simulink model "AcO_Ctrl_Geometric_headless_R2016a"  (R2016a)
settings: Solver=FixedStepDiscrete  StartTime=0.0  StopTime=simulation_duration  FixedStep=Ts  RelTol=1e-3
values from neighbouring files (symbols this model uses):
  M1_BeMo_d = zeros(7,M1_n_mode)    [AcO_Ctrl_headless_cfg.m]    (also in agws_cfg.m = 1e-6*bsxfun(@times,randn(7,M1_n_mode),scale); agws_fastTT_cfg.m = 1e-6*bsxfun(@times,randn(7,M1_n_mode),scale))
  M1_RiBo_d = zeros(7,6)    [AcO_Ctrl_headless_cfg.m]    (also in agws_cfg.m = [M1_Txyz0 M1_Rxyz0]; agws_fastTT_cfg.m = [M1_Txyz0 M1_Rxyz0])
  M2_RiBo_d = zeros(7,6)    [AcO_Ctrl_headless_cfg.m]    (also in agws_cfg.m = [M2_Txyz0 M2_Rxyz0]; agws_fastTT_cfg.m = [M2_Txyz0 M2_Rxyz0])
  Ts = 1/fs    (= 0.002)    [AcO_Ctrl_headless_cfg.m]    (also in agws_fastTT_cfg.m = 0.005)
undefined symbols (not defined in the file or in its folder): Az_C, CG2Hp, CG2Hp_S7, El_C, Fsmm, GIR_C, Hp2CG_f, Hp2CG_f_S7, HPdtf, HpK, KM2, M2_actdyn, M2_CG2Hp, M_LOS, MIMO_C, PTT2act, PTT2act_even, Q, sysd, TT2act, TT2act_even
undefined symbols (not defined in the file): on_axis_src_outputs
libraries: CEO x2
(part 3 of 6)

== system AcO_Ctrl_Geometric_headless_R2016a/Structural Dynamics V3.3/Structural Dynamics V3.3/Structural Dynamics Plus CL Az El M1 force/Az Control ==
  In1 : Inport
  -1(2) : Gain  Gain=-ones(4,1)  Multiplication=Matrix(K*u)
  Azimuth Controller : DiscreteFilter  Numerator=Az_C.num{1}  Denominator=Az_C.den{1}  SampleTime=1/500
  DEMUX1 : Gain  Gain=ones(4,1)  Multiplication=Matrix(K*u)
  Out1 : Outport
  Out2 : Outport  Port=2
  wires:
  -1(2)/1 -> Out2/1
  Azimuth Controller/1 -> DEMUX1/1, -1(2)/1
  DEMUX1/1 -> Out1/1
  In1/1 -> Azimuth Controller/1

== system AcO_Ctrl_Geometric_headless_R2016a/Structural Dynamics V3.3/Structural Dynamics V3.3/Structural Dynamics Plus CL Az El M1 force/Az El Sensing ==
  note: Note: units are m, not radians for these loops!
      | These loops delta the top and bottom displacements in tangential direction, and average the results.
  Az_top_disp(4) : Inport
  El_bottom_disp(4) : Inport  Port=2
  El_top_disp(4) : Inport  Port=3
  Az_bot_disp(4) : Inport  Port=4
  Az : Scope
  El : Scope
  Sum2 : Sum  Inputs=-+|
  Sum3 : Sum  Inputs=-+|
  average : Gain  Gain=ones(1,4)/4  Multiplication=Matrix(K*u)
  average1 : Gain  Gain=ones(1,4)/4  Multiplication=Matrix(K*u)
  El_average(1) : Outport
  Az_average(1) : Outport  Port=2
  wires:
  El_top_disp(4)/1 -> Sum2/2
  El_bottom_disp(4)/1 -> Sum2/1
  Sum2/1 -> average/1
  Sum3/1 -> average1/1
  average1/1 -> Az/1, Az_average(1)/1
  Az_bot_disp(4)/1 -> Sum3/1
  Az_top_disp(4)/1 -> Sum3/2
  average/1 -> El_average(1)/1, El/1

== system AcO_Ctrl_Geometric_headless_R2016a/Structural Dynamics V3.3/Structural Dynamics V3.3/Structural Dynamics Plus CL Az El M1 force/El Control ==
  In1 : Inport
  -1 : Gain  Gain=-ones(4,1)  Multiplication=Matrix(K*u)
  DEMUX : Gain  Gain=ones(4,1)  Multiplication=Matrix(K*u)
  Elevation Controller : DiscreteFilter  Numerator=El_C.num{1}  Denominator=El_C.den{1}  SampleTime=1/500
  Out1 : Outport
  Out2 : Outport  Port=2
  wires:
  In1/1 -> Elevation Controller/1
  DEMUX/1 -> Out2/1
  -1/1 -> Out1/1
  Elevation Controller/1 -> DEMUX/1, -1/1

== system AcO_Ctrl_Geometric_headless_R2016a/Structural Dynamics V3.3/Structural Dynamics V3.3/Structural Dynamics Plus CL Az El M1 force/M1 Displacement Local Control ==
  note: Offset displacement, used
      | in calcuation of hard point
      | forces.
  note: Hexapod Offset Forces
  note: Hexapod Desired Lengths
  note: This block converts from CG displacements and rotations,
      | and converts to Hard Point lengths.  Hard point lengths are
      | changed by applying an equal and opposite force to the hard
      | point, and then offseting output by the commanded change
      | in position.
  note: CG desired displacement/rotation
  M1_cmd(42) : Inport
  CG2Hp{1..6} (6 alike) : Gain  Gain=CG2Hp  Multiplication=Matrix(K*u)
  CG2Hp7 : Gain  Gain=CG2Hp_S7  Multiplication=Matrix(K*u)
  Demux1 : Demux  Outputs=6*ones(7,1)
  HpK{1,3..8} (7 alike) : Gain  Gain=HpK  Multiplication=Matrix(K*u)
  Mux1 : Mux  Inputs=6*ones(7,1)
  Mux3 : Mux  Inputs=6*ones(7,1)
  M1_HP_D_cmd(42) : Outport
  M1_HP_F_cmd (42) : Outport  Port=2
  wires:
  HpK8/1 -> Mux3/1
  CG2Hp7/1 -> Mux1/1, HpK8/1
  Demux1/1 -> CG2Hp7/1
  Demux1/7 -> CG2Hp6/1
  Demux1/6 -> CG2Hp5/1
  Demux1/5 -> CG2Hp4/1
  Demux1/4 -> CG2Hp3/1
  Demux1/3 -> CG2Hp2/1
  HpK7/1 -> Mux3/7
  HpK6/1 -> Mux3/6
  HpK5/1 -> Mux3/5
  HpK4/1 -> Mux3/4
  HpK1/1 -> Mux3/3
  CG2Hp6/1 -> HpK7/1, Mux1/7
  CG2Hp5/1 -> HpK6/1, Mux1/6
  CG2Hp4/1 -> HpK5/1, Mux1/5
  CG2Hp3/1 -> HpK4/1, Mux1/4
  CG2Hp2/1 -> Mux1/3, HpK1/1
  CG2Hp1/1 -> HpK3/1, Mux1/2
  Demux1/2 -> CG2Hp1/1
  M1_cmd(42)/1 -> Demux1/1
  Mux1/1 -> M1_HP_D_cmd(42)/1
  Mux3/1 -> M1_HP_F_cmd (42)/1
  HpK3/1 -> Mux3/2

== system AcO_Ctrl_Geometric_headless_R2016a/Structural Dynamics V3.3/Structural Dynamics V3.3/Structural Dynamics Plus CL Az El M1 force/M1 Force Control ==
  note: Face Forces (N)
  note: Cell Forces (N)
  note: in Newtons
  M1_measured_Force(42) : Inport
  ControlM1S1 : Subsystem
  ControlM1S2 : Subsystem
  ControlM1S3 : Subsystem
  ControlM1S4 : Subsystem
  ControlM1S5 : Subsystem
  ControlM1S6 : Subsystem
  ControlM1S7 : Subsystem
  Demux3 : Demux  Outputs=6*ones(7,1)
  M1S7 FaceForce : Outport
  M1S1 FaceForce : Outport  Port=2
  M1S2 FaceForce : Outport  Port=3
  M1S3 FaceForce : Outport  Port=4
  M1S4 FaceForce : Outport  Port=5
  M1S5 FaceForce : Outport  Port=6
  M1S6 FaceForce : Outport  Port=7
  M1S7 CellForce : Outport  Port=8
  M1S1 CellForce : Outport  Port=9
  M1S2 CellForce : Outport  Port=10
  M1S3 CellForce : Outport  Port=11
  M1S4 CellForce : Outport  Port=12
  M1S5 CellForce : Outport  Port=13
  M1S6 CellForce : Outport  Port=14
  wires:
  ControlM1S7/2(Out2) -> M1S7 CellForce/1
  ControlM1S7/1(Out1) -> M1S7 FaceForce/1
  Demux3/1 -> ControlM1S7/1(In1)
  ControlM1S6/2(Out2) -> M1S6 CellForce/1
  ControlM1S5/2(Out2) -> M1S5 CellForce/1
  ControlM1S4/2(Out2) -> M1S4 CellForce/1
  ControlM1S3/2(Out2) -> M1S3 CellForce/1
  ControlM1S2/2(Out2) -> M1S2 CellForce/1
  ControlM1S6/1(Out1) -> M1S6 FaceForce/1
  ControlM1S5/1(Out1) -> M1S5 FaceForce/1
  ControlM1S4/1(Out1) -> M1S4 FaceForce/1
  ControlM1S3/1(Out1) -> M1S3 FaceForce/1
  ControlM1S2/1(Out1) -> M1S2 FaceForce/1
  Demux3/7 -> ControlM1S6/1(In1)
  Demux3/6 -> ControlM1S5/1(In1)
  Demux3/5 -> ControlM1S4/1(In1)
  Demux3/4 -> ControlM1S3/1(In1)
  Demux3/3 -> ControlM1S2/1(In1)
  Demux3/2 -> ControlM1S1/1(In1)
  ControlM1S1/1(Out1) -> M1S1 FaceForce/1
  ControlM1S1/2(Out2) -> M1S1 CellForce/1
  M1_measured_Force(42)/1 -> Demux3/1

== system AcO_Ctrl_Geometric_headless_R2016a/Structural Dynamics V3.3/Structural Dynamics V3.3/Structural Dynamics Plus CL Az El M1 force/M1 Sensing ==
  M1_cmd (42) : Inport
  M1_HP_cell(42) : Inport  Port=2
  M1_HPface(42) : Inport  Port=3
  Demux1 : Demux  Outputs=6*ones(7,1)
  Demux2 : Demux  Outputs=6*ones(7,1)
  Demux9 : Demux  Outputs=6*ones(7,1)
  Mux3 : Mux  Inputs=6*ones(7,1)
  Scope : Scope
  Scope1 : Scope
  senseM1S1 : Subsystem
  senseM1S2 : Subsystem
  senseM1S3 : Subsystem
  senseM1S4 : Subsystem
  senseM1S5 : Subsystem
  senseM1S6 : Subsystem
  senseM1S7 : Subsystem
  M1 Hard Point Force(42) : Outport
  wires:
  M1_HPface(42)/1 -> Demux1/1
  Demux9/7 -> senseM1S6/1(HP_D_cmd)
  Demux9/5 -> senseM1S4/1(HP_D_cmd)
  Demux9/1 -> senseM1S7/1(HP_D_cmd)
  Demux9/6 -> senseM1S5/1(HP_D_cmd)
  Demux9/4 -> senseM1S3/1(HP_D_cmd)
  M1_cmd (42)/1 -> Demux9/1
  Demux9/3 -> senseM1S2/1(HP_D_cmd)
  Demux1/3 -> senseM1S2/2(HP_D_face)
  Demux1/2 -> senseM1S1/2(HP_D_face), Scope1/1
  Demux9/2 -> senseM1S1/1(HP_D_cmd)
  Mux3/1 -> M1 Hard Point Force(42)/1
  senseM1S6/1(HardPoint_6DOF_Force) -> Mux3/7
  Demux1/6 -> senseM1S5/2(HP_D_face)
  Demux1/7 -> senseM1S6/2(HP_D_face)
  Demux2/1 -> senseM1S7/3(HP_D_cell)
  M1_HP_cell(42)/1 -> Demux2/1
  senseM1S2/1(HardPoint_6DOF_Force) -> Mux3/3
  senseM1S3/1(HardPoint_6DOF_Force) -> Mux3/4
  senseM1S4/1(HardPoint_6DOF_Force) -> Mux3/5
  Demux1/1 -> senseM1S7/2(HP_D_face)
  Demux2/6 -> senseM1S5/3(HP_D_cell)
  Demux2/7 -> senseM1S6/3(HP_D_cell)
  senseM1S7/1(HardPoint_6DOF_Force) -> Mux3/1
  senseM1S5/1(HardPoint_6DOF_Force) -> Mux3/6
  Demux1/5 -> senseM1S4/2(HP_D_face)
  Demux2/4 -> senseM1S3/3(HP_D_cell)
  Demux2/3 -> senseM1S2/3(HP_D_cell)
  Demux2/2 -> senseM1S1/3(HP_D_cell)
  senseM1S1/1(HardPoint_6DOF_Force) -> Mux3/2, Scope/1
  Demux1/4 -> senseM1S3/2(HP_D_face)
  Demux2/5 -> senseM1S4/3(HP_D_cell)

== system AcO_Ctrl_Geometric_headless_R2016a/Structural Dynamics V3.3/Structural Dynamics V3.3/Structural Dynamics Plus CL Az El M1 force/M2 control ==
  note: fancy way of outputting equal and opposite forces
  note: TT command (radians)
  note: This one is grouped differently so that it is clear that odds and evens are slightly different.
      | Each subsystem controller includes both the TT controller from TT command, to PZT position command, to PZT force (using an open loop approximation).
  note: in radians
  note: in Newtons
  note: Convert from PTT to actuator
      | DOF
  note: M2 actuator Dynamics
  PTT ref (21) : Inport
  Demux1 : Demux  Outputs=3*ones(7,1)
  M2actuatorDyanmics{1..7} (7 alike) : DiscreteStateSpace  A=M2_actdyn.A  B=M2_actdyn.B  C=M2_actdyn.C  D=M2_actdyn.D  SampleTime=1/Fsmm
  TT_to_act{,1..3} (4 alike) : Gain  Gain=PTT2act  Multiplication=Matrix(K*u)
  TT_to_act4 : Gain  Gain=PTT2act_even  Multiplication=Matrix(K*u)
  TT_to_act5 : Gain  Gain=PTT2act_even  Multiplication=Matrix(K*u)
  TT_to_act6 : Gain  Gain=PTT2act_even  Multiplication=Matrix(K*u)
  delta{2..8} (7 alike) : Gain  Gain=[eye(3);-eye(3)]  Multiplication=Matrix(K*u)
  M2S7PZT_F : Outport
  M2S1PZT_F : Outport  Port=2
  M2S2PZT_F : Outport  Port=3
  M2S3PZT_F : Outport  Port=4
  M2S4PZT_F : Outport  Port=5
  M2S5PZT_F : Outport  Port=6
  M2S6PZT_F : Outport  Port=7
  wires:
  PTT ref (21)/1 -> Demux1/1
  delta5/1 -> M2S3PZT_F/1
  delta3/1 -> M2S1PZT_F/1
  TT_to_act6/1 -> M2actuatorDyanmics7/1
  M2actuatorDyanmics7/1 -> delta8/1
  TT_to_act3/1 -> M2actuatorDyanmics6/1
  M2actuatorDyanmics6/1 -> delta7/1
  TT_to_act5/1 -> M2actuatorDyanmics5/1
  M2actuatorDyanmics5/1 -> delta6/1
  TT_to_act2/1 -> M2actuatorDyanmics4/1
  M2actuatorDyanmics4/1 -> delta5/1
  TT_to_act4/1 -> M2actuatorDyanmics3/1
  M2actuatorDyanmics3/1 -> delta4/1
  TT_to_act1/1 -> M2actuatorDyanmics2/1
  M2actuatorDyanmics2/1 -> delta3/1
  TT_to_act/1 -> M2actuatorDyanmics1/1
  M2actuatorDyanmics1/1 -> delta2/1
  delta8/1 -> M2S6PZT_F/1
  delta7/1 -> M2S5PZT_F/1
  delta6/1 -> M2S4PZT_F/1
  delta4/1 -> M2S2PZT_F/1
  delta2/1 -> M2S7PZT_F/1
  Demux1/1 -> TT_to_act/1
  Demux1/7 -> TT_to_act6/1
  Demux1/6 -> TT_to_act3/1
  Demux1/5 -> TT_to_act5/1
  Demux1/4 -> TT_to_act2/1
  Demux1/3 -> TT_to_act4/1
  Demux1/2 -> TT_to_act1/1

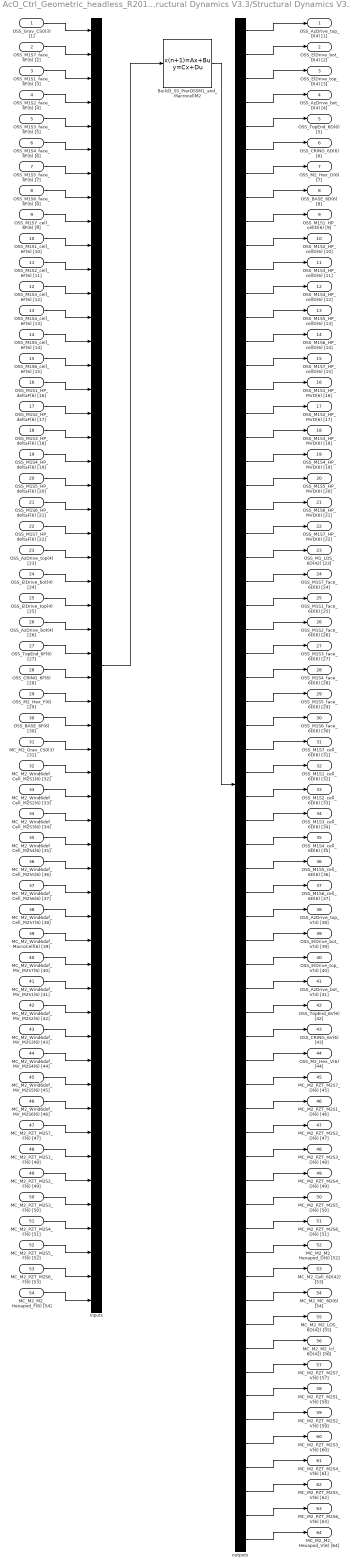
== system AcO_Ctrl_Geometric_headless_R2016a/Structural Dynamics V3.3/Structural Dynamics V3.3/Structural Dynamics Plus CL Az El M1 force/PlantDynamics Build3_SS_PierOSSM1_and_MacrocellM2 ==
  OSS_Grav_CS0(3) [1] : Inport  PortDimensions=3
  OSS_M1S7_face_6F(6) [2] : Inport  Port=2  PortDimensions=6
  OSS_M1S1_face_6F(6) [3] : Inport  Port=3  PortDimensions=6
  OSS_M1S2_face_6F(6) [4] : Inport  Port=4  PortDimensions=6
  OSS_M1S3_face_6F(6) [5] : Inport  Port=5  PortDimensions=6
  OSS_M1S4_face_6F(6) [6] : Inport  Port=6  PortDimensions=6
  OSS_M1S5_face_6F(6) [7] : Inport  Port=7  PortDimensions=6
  OSS_M1S6_face_6F(6) [8] : Inport  Port=8  PortDimensions=6
  OSS_M1S7_cell_6F(6) [9] : Inport  Port=9  PortDimensions=6
  OSS_M1S1_cell_6F(6) [10] : Inport  Port=10  PortDimensions=6
  OSS_M1S2_cell_6F(6) [11] : Inport  Port=11  PortDimensions=6
  OSS_M1S3_cell_6F(6) [12] : Inport  Port=12  PortDimensions=6
  OSS_M1S4_cell_6F(6) [13] : Inport  Port=13  PortDimensions=6
  OSS_M1S5_cell_6F(6) [14] : Inport  Port=14  PortDimensions=6
  OSS_M1S6_cell_6F(6) [15] : Inport  Port=15  PortDimensions=6
  OSS_M1S1_HP_deltaF(6) [16] : Inport  Port=16  PortDimensions=6
  OSS_M1S2_HP_deltaF(6) [17] : Inport  Port=17  PortDimensions=6
  OSS_M1S3_HP_deltaF(6) [18] : Inport  Port=18  PortDimensions=6
  OSS_M1S4_HP_deltaF(6) [19] : Inport  Port=19  PortDimensions=6
  OSS_M1S5_HP_deltaF(6) [20] : Inport  Port=20  PortDimensions=6
  OSS_M1S6_HP_deltaF(6) [21] : Inport  Port=21  PortDimensions=6
  OSS_M1S7_HP_deltaF(6) [22] : Inport  Port=22  PortDimensions=6
  OSS_AzDrive_top(4) [23] : Inport  Port=23  PortDimensions=4
  OSS_ElDrive_bot(4) [24] : Inport  Port=24  PortDimensions=4
  OSS_ElDrive_top(4) [25] : Inport  Port=25  PortDimensions=4
  OSS_AzDrive_bot(4) [26] : Inport  Port=26  PortDimensions=4
  OSS_TopEnd_6F(6) [27] : Inport  Port=27  PortDimensions=6
  OSS_CRING_6F(6) [28] : Inport  Port=28  PortDimensions=6
  OSS_M2_Hex_F(6) [29] : Inport  Port=29  PortDimensions=6
  OSS_BASE_6F(6) [30] : Inport  Port=30  PortDimensions=6
  MC_M2_Grav_CS0(3) [31] : Inport  Port=31  PortDimensions=3
  MC_M2_Wind6dof_Cell_M2S1(6) [32] : Inport  Port=32  PortDimensions=6
  MC_M2_Wind6dof_Cell_M2S2(6) [33] : Inport  Port=33  PortDimensions=6
  MC_M2_Wind6dof_Cell_M2S3(6) [34] : Inport  Port=34  PortDimensions=6
  MC_M2_Wind6dof_Cell_M2S4(6) [35] : Inport  Port=35  PortDimensions=6
  MC_M2_Wind6dof_Cell_M2S5(6) [36] : Inport  Port=36  PortDimensions=6
  MC_M2_Wind6dof_Cell_M2S6(6) [37] : Inport  Port=37  PortDimensions=6
  MC_M2_Wind6dof_Cell_M2S7(6) [38] : Inport  Port=38  PortDimensions=6
  MC_M2_Wind6dof_MacroCell(6) [39] : Inport  Port=39  PortDimensions=6
  MC_M2_Wind6dof_Mir_M2S7(6) [40] : Inport  Port=40  PortDimensions=6
  MC_M2_Wind6dof_Mir_M2S1(6) [41] : Inport  Port=41  PortDimensions=6
  MC_M2_Wind6dof_Mir_M2S2(6) [42] : Inport  Port=42  PortDimensions=6
  MC_M2_Wind6dof_Mir_M2S3(6) [43] : Inport  Port=43  PortDimensions=6
  MC_M2_Wind6dof_Mir_M2S4(6) [44] : Inport  Port=44  PortDimensions=6
  MC_M2_Wind6dof_Mir_M2S5(6) [45] : Inport  Port=45  PortDimensions=6
  MC_M2_Wind6dof_Mir_M2S6(6) [46] : Inport  Port=46  PortDimensions=6
  MC_M2_PZT_M2S7_F(6) [47] : Inport  Port=47  PortDimensions=6
  MC_M2_PZT_M2S1_F(6) [48] : Inport  Port=48  PortDimensions=6
  MC_M2_PZT_M2S2_F(6) [49] : Inport  Port=49  PortDimensions=6
  MC_M2_PZT_M2S3_F(6) [50] : Inport  Port=50  PortDimensions=6
  MC_M2_PZT_M2S4_F(6) [51] : Inport  Port=51  PortDimensions=6
  MC_M2_PZT_M2S5_F(6) [52] : Inport  Port=52  PortDimensions=6
  MC_M2_PZT_M2S6_F(6) [53] : Inport  Port=53  PortDimensions=6
  MC_M2_M2_Hexapod_F(6) [54] : Inport  Port=54  PortDimensions=6
  Build3_SS_PierOSSM1_and_MacrocellM2 : DiscreteStateSpace  A=sysd.sys.A  B=sysd.sys.B  C=sysd.sys.C  D=sysd.sys.D  SampleTime=0.002
  inputs : Mux  Inputs=[3,6,6,6,6,6,6,6,6,6,6,6,6,6,6,6,6,6,6,6,6,6,4,4,4,4,6,6,6,6,3,6,6,6,6,6,6,6,6,6,6,6,6,6,6,6,6,6,6,6,6,6,6,6]
  outputs : Demux  Outputs=[4,4,4,4,6,6,6,6,6,6,6,6,6,6,6,6,6,6,6,6,6,6,42,6,6,6,6,6,6,6,6,6,6,6,6,6,6,4,4,4,4,6,6,6,6,6,6,6,6,6,6,6,42,6,42,42,6,6,6,6,6,6,6,6]
  OSS_AzDrive_top_D(4) [1] : Outport  PortDimensions=4
  OSS_ElDrive_bot_D(4) [2] : Outport  Port=2  PortDimensions=4
  OSS_ElDrive_top_D(4) [3] : Outport  Port=3  PortDimensions=4
  OSS_AzDrive_bot_D(4) [4] : Outport  Port=4  PortDimensions=4
  OSS_TopEnd_6D(6) [5] : Outport  Port=5  PortDimensions=6
  OSS_CRING_6D(6) [6] : Outport  Port=6  PortDimensions=6
  OSS_M2_Hex_D(6) [7] : Outport  Port=7  PortDimensions=6
  OSS_BASE_6D(6) [8] : Outport  Port=8  PortDimensions=6
  OSS_M1S1_HP_cellD(6) [9] : Outport  Port=9  PortDimensions=6
  OSS_M1S2_HP_cellD(6) [10] : Outport  Port=10  PortDimensions=6
  OSS_M1S3_HP_cellD(6) [11] : Outport  Port=11  PortDimensions=6
  OSS_M1S4_HP_cellD(6) [12] : Outport  Port=12  PortDimensions=6
  OSS_M1S5_HP_cellD(6) [13] : Outport  Port=13  PortDimensions=6
  OSS_M1S6_HP_cellD(6) [14] : Outport  Port=14  PortDimensions=6
  OSS_M1S7_HP_cellD(6) [15] : Outport  Port=15  PortDimensions=6
  OSS_M1S1_HP_MirD(6) [16] : Outport  Port=16  PortDimensions=6
  OSS_M1S2_HP_MirD(6) [17] : Outport  Port=17  PortDimensions=6
  OSS_M1S3_HP_MirD(6) [18] : Outport  Port=18  PortDimensions=6
  OSS_M1S4_HP_MirD(6) [19] : Outport  Port=19  PortDimensions=6
  OSS_M1S5_HP_MirD(6) [20] : Outport  Port=20  PortDimensions=6
  OSS_M1S6_HP_MirD(6) [21] : Outport  Port=21  PortDimensions=6
  OSS_M1S7_HP_MirD(6) [22] : Outport  Port=22  PortDimensions=6
  OSS_M1_LOS_6D(42) [23] : Outport  Port=23  PortDimensions=42
  OSS_M1S7_face_6D(6) [24] : Outport  Port=24  PortDimensions=6
  OSS_M1S1_face_6D(6) [25] : Outport  Port=25  PortDimensions=6
  OSS_M1S2_face_6D(6) [26] : Outport  Port=26  PortDimensions=6
  OSS_M1S3_face_6D(6) [27] : Outport  Port=27  PortDimensions=6
  OSS_M1S4_face_6D(6) [28] : Outport  Port=28  PortDimensions=6
  OSS_M1S5_face_6D(6) [29] : Outport  Port=29  PortDimensions=6
  OSS_M1S6_face_6D(6) [30] : Outport  Port=30  PortDimensions=6
  OSS_M1S7_cell_6D(6) [31] : Outport  Port=31  PortDimensions=6
  OSS_M1S1_cell_6D(6) [32] : Outport  Port=32  PortDimensions=6
  OSS_M1S2_cell_6D(6) [33] : Outport  Port=33  PortDimensions=6
  OSS_M1S3_cell_6D(6) [34] : Outport  Port=34  PortDimensions=6
  OSS_M1S4_cell_6D(6) [35] : Outport  Port=35  PortDimensions=6
  OSS_M1S5_cell_6D(6) [36] : Outport  Port=36  PortDimensions=6
  OSS_M1S6_cell_6D(6) [37] : Outport  Port=37  PortDimensions=6
  OSS_AzDrive_top_V(4) [38] : Outport  Port=38  PortDimensions=4
  OSS_ElDrive_bot_V(4) [39] : Outport  Port=39  PortDimensions=4
  OSS_ElDrive_top_V(4) [40] : Outport  Port=40  PortDimensions=4
  OSS_AzDrive_bot_V(4) [41] : Outport  Port=41  PortDimensions=4
  OSS_TopEnd_6V(6) [42] : Outport  Port=42  PortDimensions=6
  OSS_CRING_6V(6) [43] : Outport  Port=43  PortDimensions=6
  OSS_M2_Hex_V(6) [44] : Outport  Port=44  PortDimensions=6
  MC_M2_PZT_M2S7_D(6) [45] : Outport  Port=45  PortDimensions=6
  MC_M2_PZT_M2S1_D(6) [46] : Outport  Port=46  PortDimensions=6
  MC_M2_PZT_M2S2_D(6) [47] : Outport  Port=47  PortDimensions=6
  MC_M2_PZT_M2S3_D(6) [48] : Outport  Port=48  PortDimensions=6
  MC_M2_PZT_M2S4_D(6) [49] : Outport  Port=49  PortDimensions=6
  MC_M2_PZT_M2S5_D(6) [50] : Outport  Port=50  PortDimensions=6
  MC_M2_PZT_M2S6_D(6) [51] : Outport  Port=51  PortDimensions=6
  MC_M2_M2_Hexapod_D(6) [52] : Outport  Port=52  PortDimensions=6
  MC_M2_Cell_6D(42) [53] : Outport  Port=53  PortDimensions=42
  MC_M2_MC_6D(6) [54] : Outport  Port=54  PortDimensions=6
  MC_M2_M2_LOS_6D(42) [55] : Outport  Port=55  PortDimensions=42
  MC_M2_M2_lcl_6D(42) [56] : Outport  Port=56  PortDimensions=42
  MC_M2_PZT_M2S7_V(6) [57] : Outport  Port=57  PortDimensions=6
  MC_M2_PZT_M2S1_V(6) [58] : Outport  Port=58  PortDimensions=6
  MC_M2_PZT_M2S2_V(6) [59] : Outport  Port=59  PortDimensions=6
  MC_M2_PZT_M2S3_V(6) [60] : Outport  Port=60  PortDimensions=6
  MC_M2_PZT_M2S4_V(6) [61] : Outport  Port=61  PortDimensions=6
  MC_M2_PZT_M2S5_V(6) [62] : Outport  Port=62  PortDimensions=6
  MC_M2_PZT_M2S6_V(6) [63] : Outport  Port=63  PortDimensions=6
  MC_M2_M2_Hexapod_V(6) [64] : Outport  Port=64  PortDimensions=6
  wires:
  outputs/64 -> MC_M2_M2_Hexapod_V(6) [64]/1
  outputs/63 -> MC_M2_PZT_M2S6_V(6) [63]/1
  outputs/62 -> MC_M2_PZT_M2S5_V(6) [62]/1
  outputs/61 -> MC_M2_PZT_M2S4_V(6) [61]/1
  outputs/60 -> MC_M2_PZT_M2S3_V(6) [60]/1
  outputs/59 -> MC_M2_PZT_M2S2_V(6) [59]/1
  outputs/58 -> MC_M2_PZT_M2S1_V(6) [58]/1
  outputs/57 -> MC_M2_PZT_M2S7_V(6) [57]/1
  outputs/56 -> MC_M2_M2_lcl_6D(42) [56]/1
  outputs/55 -> MC_M2_M2_LOS_6D(42) [55]/1
  outputs/54 -> MC_M2_MC_6D(6) [54]/1
  outputs/53 -> MC_M2_Cell_6D(42) [53]/1
  outputs/52 -> MC_M2_M2_Hexapod_D(6) [52]/1
  outputs/51 -> MC_M2_PZT_M2S6_D(6) [51]/1
  outputs/50 -> MC_M2_PZT_M2S5_D(6) [50]/1
  outputs/49 -> MC_M2_PZT_M2S4_D(6) [49]/1
  outputs/48 -> MC_M2_PZT_M2S3_D(6) [48]/1
  outputs/47 -> MC_M2_PZT_M2S2_D(6) [47]/1
  outputs/46 -> MC_M2_PZT_M2S1_D(6) [46]/1
  outputs/45 -> MC_M2_PZT_M2S7_D(6) [45]/1
  outputs/44 -> OSS_M2_Hex_V(6) [44]/1
  outputs/43 -> OSS_CRING_6V(6) [43]/1
  outputs/42 -> OSS_TopEnd_6V(6) [42]/1
  outputs/41 -> OSS_AzDrive_bot_V(4) [41]/1
  outputs/40 -> OSS_ElDrive_top_V(4) [40]/1
  outputs/39 -> OSS_ElDrive_bot_V(4) [39]/1
  outputs/38 -> OSS_AzDrive_top_V(4) [38]/1
  outputs/37 -> OSS_M1S6_cell_6D(6) [37]/1
  outputs/36 -> OSS_M1S5_cell_6D(6) [36]/1
  outputs/35 -> OSS_M1S4_cell_6D(6) [35]/1
  outputs/34 -> OSS_M1S3_cell_6D(6) [34]/1
  outputs/33 -> OSS_M1S2_cell_6D(6) [33]/1
  outputs/32 -> OSS_M1S1_cell_6D(6) [32]/1
  outputs/31 -> OSS_M1S7_cell_6D(6) [31]/1
  outputs/30 -> OSS_M1S6_face_6D(6) [30]/1
  outputs/29 -> OSS_M1S5_face_6D(6) [29]/1
  outputs/28 -> OSS_M1S4_face_6D(6) [28]/1
  outputs/27 -> OSS_M1S3_face_6D(6) [27]/1
  outputs/26 -> OSS_M1S2_face_6D(6) [26]/1
  outputs/25 -> OSS_M1S1_face_6D(6) [25]/1
  outputs/24 -> OSS_M1S7_face_6D(6) [24]/1
  outputs/23 -> OSS_M1_LOS_6D(42) [23]/1
  outputs/22 -> OSS_M1S7_HP_MirD(6) [22]/1
  outputs/21 -> OSS_M1S6_HP_MirD(6) [21]/1
  outputs/20 -> OSS_M1S5_HP_MirD(6) [20]/1
  outputs/19 -> OSS_M1S4_HP_MirD(6) [19]/1
  outputs/18 -> OSS_M1S3_HP_MirD(6) [18]/1
  outputs/17 -> OSS_M1S2_HP_MirD(6) [17]/1
  outputs/16 -> OSS_M1S1_HP_MirD(6) [16]/1
  outputs/15 -> OSS_M1S7_HP_cellD(6) [15]/1
  outputs/14 -> OSS_M1S6_HP_cellD(6) [14]/1
  outputs/13 -> OSS_M1S5_HP_cellD(6) [13]/1
  outputs/12 -> OSS_M1S4_HP_cellD(6) [12]/1
  outputs/11 -> OSS_M1S3_HP_cellD(6) [11]/1
  outputs/10 -> OSS_M1S2_HP_cellD(6) [10]/1
  outputs/9 -> OSS_M1S1_HP_cellD(6) [9]/1
  outputs/8 -> OSS_BASE_6D(6) [8]/1
  outputs/7 -> OSS_M2_Hex_D(6) [7]/1
  outputs/6 -> OSS_CRING_6D(6) [6]/1
  outputs/5 -> OSS_TopEnd_6D(6) [5]/1
  outputs/4 -> OSS_AzDrive_bot_D(4) [4]/1
  outputs/3 -> OSS_ElDrive_top_D(4) [3]/1
  outputs/2 -> OSS_ElDrive_bot_D(4) [2]/1
  outputs/1 -> OSS_AzDrive_top_D(4) [1]/1
  Build3_SS_PierOSSM1_and_MacrocellM2/1 -> outputs/1
  inputs/1 -> Build3_SS_PierOSSM1_and_MacrocellM2/1
  MC_M2_M2_Hexapod_F(6) [54]/1 -> inputs/54
  MC_M2_PZT_M2S6_F(6) [53]/1 -> inputs/53
  MC_M2_PZT_M2S5_F(6) [52]/1 -> inputs/52
  MC_M2_PZT_M2S4_F(6) [51]/1 -> inputs/51
  MC_M2_PZT_M2S3_F(6) [50]/1 -> inputs/50
  MC_M2_PZT_M2S2_F(6) [49]/1 -> inputs/49
  MC_M2_PZT_M2S1_F(6) [48]/1 -> inputs/48
  MC_M2_PZT_M2S7_F(6) [47]/1 -> inputs/47
  MC_M2_Wind6dof_Mir_M2S6(6) [46]/1 -> inputs/46
  MC_M2_Wind6dof_Mir_M2S5(6) [45]/1 -> inputs/45
  MC_M2_Wind6dof_Mir_M2S4(6) [44]/1 -> inputs/44
  MC_M2_Wind6dof_Mir_M2S3(6) [43]/1 -> inputs/43
  MC_M2_Wind6dof_Mir_M2S2(6) [42]/1 -> inputs/42
  MC_M2_Wind6dof_Mir_M2S1(6) [41]/1 -> inputs/41
  MC_M2_Wind6dof_Mir_M2S7(6) [40]/1 -> inputs/40
  MC_M2_Wind6dof_MacroCell(6) [39]/1 -> inputs/39
  MC_M2_Wind6dof_Cell_M2S7(6) [38]/1 -> inputs/38
  MC_M2_Wind6dof_Cell_M2S6(6) [37]/1 -> inputs/37
  MC_M2_Wind6dof_Cell_M2S5(6) [36]/1 -> inputs/36
  MC_M2_Wind6dof_Cell_M2S4(6) [35]/1 -> inputs/35
  MC_M2_Wind6dof_Cell_M2S3(6) [34]/1 -> inputs/34
  MC_M2_Wind6dof_Cell_M2S2(6) [33]/1 -> inputs/33
  MC_M2_Wind6dof_Cell_M2S1(6) [32]/1 -> inputs/32
  MC_M2_Grav_CS0(3) [31]/1 -> inputs/31
  OSS_BASE_6F(6) [30]/1 -> inputs/30
  OSS_M2_Hex_F(6) [29]/1 -> inputs/29
  OSS_CRING_6F(6) [28]/1 -> inputs/28
  OSS_TopEnd_6F(6) [27]/1 -> inputs/27
  OSS_AzDrive_bot(4) [26]/1 -> inputs/26
  OSS_ElDrive_top(4) [25]/1 -> inputs/25
  OSS_ElDrive_bot(4) [24]/1 -> inputs/24
  OSS_AzDrive_top(4) [23]/1 -> inputs/23
  OSS_M1S7_HP_deltaF(6) [22]/1 -> inputs/22
  OSS_M1S6_HP_deltaF(6) [21]/1 -> inputs/21
  OSS_M1S5_HP_deltaF(6) [20]/1 -> inputs/20
  OSS_M1S4_HP_deltaF(6) [19]/1 -> inputs/19
  OSS_M1S3_HP_deltaF(6) [18]/1 -> inputs/18
  OSS_M1S2_HP_deltaF(6) [17]/1 -> inputs/17
  OSS_M1S1_HP_deltaF(6) [16]/1 -> inputs/16
  OSS_M1S6_cell_6F(6) [15]/1 -> inputs/15
  OSS_M1S5_cell_6F(6) [14]/1 -> inputs/14
  OSS_M1S4_cell_6F(6) [13]/1 -> inputs/13
  OSS_M1S3_cell_6F(6) [12]/1 -> inputs/12
  OSS_M1S2_cell_6F(6) [11]/1 -> inputs/11
  OSS_M1S1_cell_6F(6) [10]/1 -> inputs/10
  OSS_M1S7_cell_6F(6) [9]/1 -> inputs/9
  OSS_M1S6_face_6F(6) [8]/1 -> inputs/8
  OSS_M1S5_face_6F(6) [7]/1 -> inputs/7
  OSS_M1S4_face_6F(6) [6]/1 -> inputs/6
  OSS_M1S3_face_6F(6) [5]/1 -> inputs/5
  OSS_M1S2_face_6F(6) [4]/1 -> inputs/4
  OSS_M1S1_face_6F(6) [3]/1 -> inputs/3
  OSS_M1S7_face_6F(6) [2]/1 -> inputs/2
  OSS_Grav_CS0(3) [1]/1 -> inputs/1

== system AcO_Ctrl_Geometric_headless_R2016a/Structural Dynamics V3.3/Structural Dynamics V3.3a/Structural Dynamics Plus CL Az El M1 force/Az Control ==
  In1 : Inport
  -1(2) : Gain  Gain=-ones(4,1)  Multiplication=Matrix(K*u)
  Azimuth Controller : DiscreteFilter  Numerator=Az_C.num{1}  Denominator=Az_C.den{1}  SampleTime=1/500
  DEMUX1 : Gain  Gain=ones(4,1)  Multiplication=Matrix(K*u)
  Out1 : Outport
  Out2 : Outport  Port=2
  wires:
  In1/1 -> Azimuth Controller/1
  DEMUX1/1 -> Out1/1
  Azimuth Controller/1 -> -1(2)/1, DEMUX1/1
  -1(2)/1 -> Out2/1

== system AcO_Ctrl_Geometric_headless_R2016a/Structural Dynamics V3.3/Structural Dynamics V3.3a/Structural Dynamics Plus CL Az El M1 force/Az El Sensing ==
  note: Note: units are m, not radians for these loops!
      | These loops delta the top and bottom displacements in tangential direction, and average the results.
  Az_top_disp(4) : Inport
  El_bottom_disp(4) : Inport  Port=2
  El_top_disp(4) : Inport  Port=3
  Az_bot_disp(4) : Inport  Port=4
  Az : Scope
  El : Scope
  Sum2 : Sum  Inputs=-+|
  Sum3 : Sum  Inputs=-+|
  average : Gain  Gain=ones(1,4)/4  Multiplication=Matrix(K*u)
  average1 : Gain  Gain=ones(1,4)/4  Multiplication=Matrix(K*u)
  El_average(1) : Outport
  Az_average(1) : Outport  Port=2
  wires:
  average/1 -> El/1, El_average(1)/1
  Az_top_disp(4)/1 -> Sum3/2
  Az_bot_disp(4)/1 -> Sum3/1
  average1/1 -> Az_average(1)/1, Az/1
  Sum3/1 -> average1/1
  Sum2/1 -> average/1
  El_bottom_disp(4)/1 -> Sum2/1
  El_top_disp(4)/1 -> Sum2/2

== system AcO_Ctrl_Geometric_headless_R2016a/Structural Dynamics V3.3/Structural Dynamics V3.3a/Structural Dynamics Plus CL Az El M1 force/El Control ==
  In1 : Inport
  -1 : Gain  Gain=-ones(4,1)  Multiplication=Matrix(K*u)
  DEMUX : Gain  Gain=ones(4,1)  Multiplication=Matrix(K*u)
  Elevation Controller : DiscreteFilter  Numerator=El_C.num{1}  Denominator=El_C.den{1}  SampleTime=1/500
  Out1 : Outport
  Out2 : Outport  Port=2
  wires:
  Elevation Controller/1 -> -1/1, DEMUX/1
  -1/1 -> Out1/1
  DEMUX/1 -> Out2/1
  In1/1 -> Elevation Controller/1

== system AcO_Ctrl_Geometric_headless_R2016a/Structural Dynamics V3.3/Structural Dynamics V3.3a/Structural Dynamics Plus CL Az El M1 force/M1 Displacement Local Control ==
  note: CG desired displacement/rotation
  note: This block converts from CG displacements and rotations,
      | and converts to Hard Point lengths.  Hard point lengths are
      | changed by applying an equal and opposite force to the hard
      | point, and then offseting output by the commanded change
      | in position.
  note: Hexapod Desired Lengths
  note: Hexapod Offset Forces
  note: Offset displacement, used
      | in calcuation of hard point
      | forces.
  M1_cmd(42) : Inport
  CG2Hp{1..6} (6 alike) : Gain  Gain=CG2Hp  Multiplication=Matrix(K*u)
  CG2Hp7 : Gain  Gain=CG2Hp_S7  Multiplication=Matrix(K*u)
  Demux1 : Demux  Outputs=6*ones(7,1)
  Discrete Filter : DiscreteFilter  Numerator=HPdtf.num{1}  Denominator=HPdtf.den{1}
  HpK{1,3..8} (7 alike) : Gain  Gain=HpK  Multiplication=Matrix(K*u)
  Mux1 : Mux  Inputs=6*ones(7,1)
  Mux3 : Mux  Inputs=6*ones(7,1)
  M1_HP_D_cmd(42) : Outport
  M1_HP_F_cmd (42) : Outport  Port=2
  wires:
  HpK3/1 -> Mux3/2
  Mux3/1 -> M1_HP_F_cmd (42)/1
  Mux1/1 -> M1_HP_D_cmd(42)/1
  M1_cmd(42)/1 -> Discrete Filter/1
  Demux1/2 -> CG2Hp1/1
  CG2Hp1/1 -> Mux1/2, HpK3/1
  CG2Hp2/1 -> HpK1/1, Mux1/3
  CG2Hp3/1 -> Mux1/4, HpK4/1
  CG2Hp4/1 -> Mux1/5, HpK5/1
  CG2Hp5/1 -> Mux1/6, HpK6/1
  CG2Hp6/1 -> Mux1/7, HpK7/1
  HpK1/1 -> Mux3/3
  HpK4/1 -> Mux3/4
  HpK5/1 -> Mux3/5
  HpK6/1 -> Mux3/6
  HpK7/1 -> Mux3/7
  Demux1/3 -> CG2Hp2/1
  Demux1/4 -> CG2Hp3/1
  Demux1/5 -> CG2Hp4/1
  Demux1/6 -> CG2Hp5/1
  Demux1/7 -> CG2Hp6/1
  Demux1/1 -> CG2Hp7/1
  CG2Hp7/1 -> HpK8/1, Mux1/1
  HpK8/1 -> Mux3/1
  Discrete Filter/1 -> Demux1/1

== system AcO_Ctrl_Geometric_headless_R2016a/Structural Dynamics V3.3/Structural Dynamics V3.3a/Structural Dynamics Plus CL Az El M1 force/M1 Force Control ==
  note: in Newtons
  note: Cell Forces (N)
  note: Face Forces (N)
  M1_measured_Force(42) : Inport
  ControlM1S1 : Subsystem
  ControlM1S2 : Subsystem
  ControlM1S3 : Subsystem
  ControlM1S4 : Subsystem
  ControlM1S5 : Subsystem
  ControlM1S6 : Subsystem
  ControlM1S7 : Subsystem
  Demux3 : Demux  Outputs=6*ones(7,1)
  M1S7 FaceForce : Outport
  M1S1 FaceForce : Outport  Port=2
  M1S2 FaceForce : Outport  Port=3
  M1S3 FaceForce : Outport  Port=4
  M1S4 FaceForce : Outport  Port=5
  M1S5 FaceForce : Outport  Port=6
  M1S6 FaceForce : Outport  Port=7
  M1S7 CellForce : Outport  Port=8
  M1S1 CellForce : Outport  Port=9
  M1S2 CellForce : Outport  Port=10
  M1S3 CellForce : Outport  Port=11
  M1S4 CellForce : Outport  Port=12
  M1S5 CellForce : Outport  Port=13
  M1S6 CellForce : Outport  Port=14
  wires:
  M1_measured_Force(42)/1 -> Demux3/1
  ControlM1S1/2(Out2) -> M1S1 CellForce/1
  ControlM1S1/1(Out1) -> M1S1 FaceForce/1
  Demux3/2 -> ControlM1S1/1(In1)
  Demux3/3 -> ControlM1S2/1(In1)
  Demux3/4 -> ControlM1S3/1(In1)
  Demux3/5 -> ControlM1S4/1(In1)
  Demux3/6 -> ControlM1S5/1(In1)
  Demux3/7 -> ControlM1S6/1(In1)
  ControlM1S2/1(Out1) -> M1S2 FaceForce/1
  ControlM1S3/1(Out1) -> M1S3 FaceForce/1
  ControlM1S4/1(Out1) -> M1S4 FaceForce/1
  ControlM1S5/1(Out1) -> M1S5 FaceForce/1
  ControlM1S6/1(Out1) -> M1S6 FaceForce/1
  ControlM1S2/2(Out2) -> M1S2 CellForce/1
  ControlM1S3/2(Out2) -> M1S3 CellForce/1
  ControlM1S4/2(Out2) -> M1S4 CellForce/1
  ControlM1S5/2(Out2) -> M1S5 CellForce/1
  ControlM1S6/2(Out2) -> M1S6 CellForce/1
  Demux3/1 -> ControlM1S7/1(In1)
  ControlM1S7/1(Out1) -> M1S7 FaceForce/1
  ControlM1S7/2(Out2) -> M1S7 CellForce/1

== system AcO_Ctrl_Geometric_headless_R2016a/Structural Dynamics V3.3/Structural Dynamics V3.3a/Structural Dynamics Plus CL Az El M1 force/M1 Sensing ==
  M1_cmd (42) : Inport
  M1_HP_cell(42) : Inport  Port=2
  M1_HPface(42) : Inport  Port=3
  Demux1 : Demux  Outputs=6*ones(7,1)
  Demux2 : Demux  Outputs=6*ones(7,1)
  Demux9 : Demux  Outputs=6*ones(7,1)
  Mux3 : Mux  Inputs=6*ones(7,1)
  Scope : Scope
  Scope1 : Scope
  senseM1S1 : Subsystem
  senseM1S2 : Subsystem
  senseM1S3 : Subsystem
  senseM1S4 : Subsystem
  senseM1S5 : Subsystem
  senseM1S6 : Subsystem
  senseM1S7 : Subsystem
  M1 Hard Point Force(42) : Outport
  wires:
  Demux2/5 -> senseM1S4/3(HP_D_cell)
  Demux1/4 -> senseM1S3/2(HP_D_face)
  senseM1S1/1(HardPoint_6DOF_Force) -> Scope/1, Mux3/2
  Demux2/2 -> senseM1S1/3(HP_D_cell)
  Demux2/3 -> senseM1S2/3(HP_D_cell)
  Demux2/4 -> senseM1S3/3(HP_D_cell)
  Demux1/5 -> senseM1S4/2(HP_D_face)
  senseM1S5/1(HardPoint_6DOF_Force) -> Mux3/6
  senseM1S7/1(HardPoint_6DOF_Force) -> Mux3/1
  Demux2/7 -> senseM1S6/3(HP_D_cell)
  Demux2/6 -> senseM1S5/3(HP_D_cell)
  Demux1/1 -> senseM1S7/2(HP_D_face)
  senseM1S4/1(HardPoint_6DOF_Force) -> Mux3/5
  senseM1S3/1(HardPoint_6DOF_Force) -> Mux3/4
  senseM1S2/1(HardPoint_6DOF_Force) -> Mux3/3
  M1_HP_cell(42)/1 -> Demux2/1
  Demux2/1 -> senseM1S7/3(HP_D_cell)
  Demux1/7 -> senseM1S6/2(HP_D_face)
  Demux1/6 -> senseM1S5/2(HP_D_face)
  senseM1S6/1(HardPoint_6DOF_Force) -> Mux3/7
  Mux3/1 -> M1 Hard Point Force(42)/1
  Demux9/2 -> senseM1S1/1(HP_D_cmd)
  Demux1/2 -> Scope1/1, senseM1S1/2(HP_D_face)
  Demux1/3 -> senseM1S2/2(HP_D_face)
  Demux9/3 -> senseM1S2/1(HP_D_cmd)
  M1_cmd (42)/1 -> Demux9/1
  Demux9/4 -> senseM1S3/1(HP_D_cmd)
  Demux9/6 -> senseM1S5/1(HP_D_cmd)
  Demux9/1 -> senseM1S7/1(HP_D_cmd)
  Demux9/5 -> senseM1S4/1(HP_D_cmd)
  Demux9/7 -> senseM1S6/1(HP_D_cmd)
  M1_HPface(42)/1 -> Demux1/1

== system AcO_Ctrl_Geometric_headless_R2016a/Structural Dynamics V3.3/Structural Dynamics V3.3a/Structural Dynamics Plus CL Az El M1 force/M2 control ==
  note: M2 actuator Dynamics
  note: Convert from PTT to actuator
      | DOF
  note: in Newtons
  note: in radians
  note: This one is grouped differently so that it is clear that odds and evens are slightly different.
      | Each subsystem controller includes both the TT controller from TT command, to PZT position command, to PZT force (using an open loop approximation).
  note: TT command (radians)
  note: fancy way of outputting equal and opposite forces
  PTT ref (21) : Inport
  Demux1 : Demux  Outputs=3*ones(7,1)
  M2actuatorDyanmics{1..7} (7 alike) : DiscreteStateSpace  A=M2_actdyn.A  B=M2_actdyn.B  C=M2_actdyn.C  D=M2_actdyn.D  SampleTime=1/Fsmm
  TT_to_act{,1..3} (4 alike) : Gain  Gain=PTT2act  Multiplication=Matrix(K*u)
  TT_to_act4 : Gain  Gain=PTT2act_even  Multiplication=Matrix(K*u)
  TT_to_act5 : Gain  Gain=PTT2act_even  Multiplication=Matrix(K*u)
  TT_to_act6 : Gain  Gain=PTT2act_even  Multiplication=Matrix(K*u)
  delta{2..8} (7 alike) : Gain  Gain=[eye(3);-eye(3)]  Multiplication=Matrix(K*u)
  M2S7PZT_F : Outport
  M2S1PZT_F : Outport  Port=2
  M2S2PZT_F : Outport  Port=3
  M2S3PZT_F : Outport  Port=4
  M2S4PZT_F : Outport  Port=5
  M2S5PZT_F : Outport  Port=6
  M2S6PZT_F : Outport  Port=7
  wires:
  Demux1/2 -> TT_to_act1/1
  Demux1/3 -> TT_to_act4/1
  Demux1/4 -> TT_to_act2/1
  Demux1/5 -> TT_to_act5/1
  Demux1/6 -> TT_to_act3/1
  Demux1/7 -> TT_to_act6/1
  Demux1/1 -> TT_to_act/1
  delta2/1 -> M2S7PZT_F/1
  delta4/1 -> M2S2PZT_F/1
  delta6/1 -> M2S4PZT_F/1
  delta7/1 -> M2S5PZT_F/1
  delta8/1 -> M2S6PZT_F/1
  M2actuatorDyanmics1/1 -> delta2/1
  TT_to_act/1 -> M2actuatorDyanmics1/1
  M2actuatorDyanmics2/1 -> delta3/1
  TT_to_act1/1 -> M2actuatorDyanmics2/1
  M2actuatorDyanmics3/1 -> delta4/1
  TT_to_act4/1 -> M2actuatorDyanmics3/1
  M2actuatorDyanmics4/1 -> delta5/1
  TT_to_act2/1 -> M2actuatorDyanmics4/1
  M2actuatorDyanmics5/1 -> delta6/1
  TT_to_act5/1 -> M2actuatorDyanmics5/1
  M2actuatorDyanmics6/1 -> delta7/1
  TT_to_act3/1 -> M2actuatorDyanmics6/1
  M2actuatorDyanmics7/1 -> delta8/1
  TT_to_act6/1 -> M2actuatorDyanmics7/1
  delta3/1 -> M2S1PZT_F/1
  delta5/1 -> M2S3PZT_F/1
  PTT ref (21)/1 -> Demux1/1

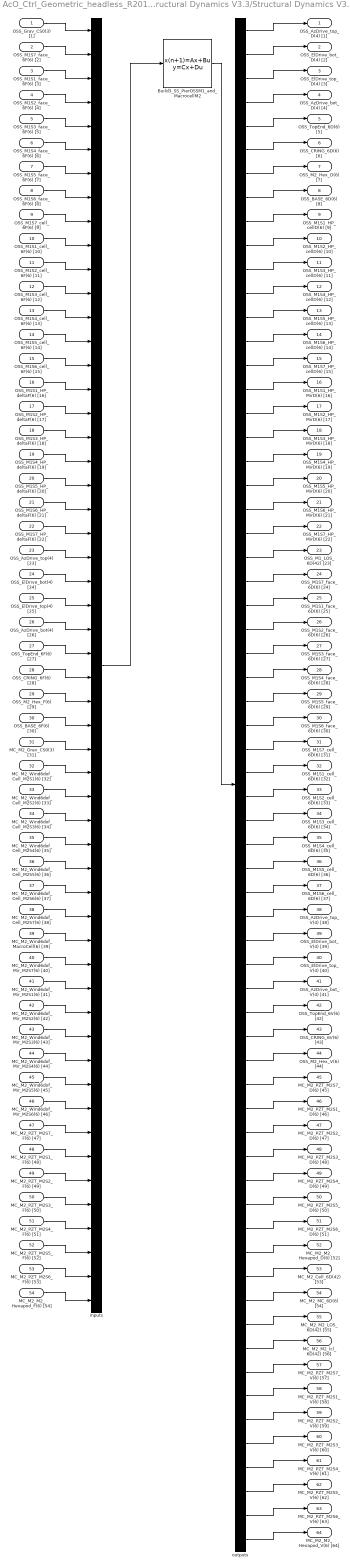
== system AcO_Ctrl_Geometric_headless_R2016a/Structural Dynamics V3.3/Structural Dynamics V3.3a/Structural Dynamics Plus CL Az El M1 force/PlantDynamics Build3_SS_PierOSSM1_and_MacrocellM2 ==
  OSS_Grav_CS0(3) [1] : Inport  PortDimensions=3
  OSS_M1S7_face_6F(6) [2] : Inport  Port=2  PortDimensions=6
  OSS_M1S1_face_6F(6) [3] : Inport  Port=3  PortDimensions=6
  OSS_M1S2_face_6F(6) [4] : Inport  Port=4  PortDimensions=6
  OSS_M1S3_face_6F(6) [5] : Inport  Port=5  PortDimensions=6
  OSS_M1S4_face_6F(6) [6] : Inport  Port=6  PortDimensions=6
  OSS_M1S5_face_6F(6) [7] : Inport  Port=7  PortDimensions=6
  OSS_M1S6_face_6F(6) [8] : Inport  Port=8  PortDimensions=6
  OSS_M1S7_cell_6F(6) [9] : Inport  Port=9  PortDimensions=6
  OSS_M1S1_cell_6F(6) [10] : Inport  Port=10  PortDimensions=6
  OSS_M1S2_cell_6F(6) [11] : Inport  Port=11  PortDimensions=6
  OSS_M1S3_cell_6F(6) [12] : Inport  Port=12  PortDimensions=6
  OSS_M1S4_cell_6F(6) [13] : Inport  Port=13  PortDimensions=6
  OSS_M1S5_cell_6F(6) [14] : Inport  Port=14  PortDimensions=6
  OSS_M1S6_cell_6F(6) [15] : Inport  Port=15  PortDimensions=6
  OSS_M1S1_HP_deltaF(6) [16] : Inport  Port=16  PortDimensions=6
  OSS_M1S2_HP_deltaF(6) [17] : Inport  Port=17  PortDimensions=6
  OSS_M1S3_HP_deltaF(6) [18] : Inport  Port=18  PortDimensions=6
  OSS_M1S4_HP_deltaF(6) [19] : Inport  Port=19  PortDimensions=6
  OSS_M1S5_HP_deltaF(6) [20] : Inport  Port=20  PortDimensions=6
  OSS_M1S6_HP_deltaF(6) [21] : Inport  Port=21  PortDimensions=6
  OSS_M1S7_HP_deltaF(6) [22] : Inport  Port=22  PortDimensions=6
  OSS_AzDrive_top(4) [23] : Inport  Port=23  PortDimensions=4
  OSS_ElDrive_bot(4) [24] : Inport  Port=24  PortDimensions=4
  OSS_ElDrive_top(4) [25] : Inport  Port=25  PortDimensions=4
  OSS_AzDrive_bot(4) [26] : Inport  Port=26  PortDimensions=4
  OSS_TopEnd_6F(6) [27] : Inport  Port=27  PortDimensions=6
  OSS_CRING_6F(6) [28] : Inport  Port=28  PortDimensions=6
  OSS_M2_Hex_F(6) [29] : Inport  Port=29  PortDimensions=6
  OSS_BASE_6F(6) [30] : Inport  Port=30  PortDimensions=6
  MC_M2_Grav_CS0(3) [31] : Inport  Port=31  PortDimensions=3
  MC_M2_Wind6dof_Cell_M2S1(6) [32] : Inport  Port=32  PortDimensions=6
  MC_M2_Wind6dof_Cell_M2S2(6) [33] : Inport  Port=33  PortDimensions=6
  MC_M2_Wind6dof_Cell_M2S3(6) [34] : Inport  Port=34  PortDimensions=6
  MC_M2_Wind6dof_Cell_M2S4(6) [35] : Inport  Port=35  PortDimensions=6
  MC_M2_Wind6dof_Cell_M2S5(6) [36] : Inport  Port=36  PortDimensions=6
  MC_M2_Wind6dof_Cell_M2S6(6) [37] : Inport  Port=37  PortDimensions=6
  MC_M2_Wind6dof_Cell_M2S7(6) [38] : Inport  Port=38  PortDimensions=6
  MC_M2_Wind6dof_MacroCell(6) [39] : Inport  Port=39  PortDimensions=6
  MC_M2_Wind6dof_Mir_M2S7(6) [40] : Inport  Port=40  PortDimensions=6
  MC_M2_Wind6dof_Mir_M2S1(6) [41] : Inport  Port=41  PortDimensions=6
  MC_M2_Wind6dof_Mir_M2S2(6) [42] : Inport  Port=42  PortDimensions=6
  MC_M2_Wind6dof_Mir_M2S3(6) [43] : Inport  Port=43  PortDimensions=6
  MC_M2_Wind6dof_Mir_M2S4(6) [44] : Inport  Port=44  PortDimensions=6
  MC_M2_Wind6dof_Mir_M2S5(6) [45] : Inport  Port=45  PortDimensions=6
  MC_M2_Wind6dof_Mir_M2S6(6) [46] : Inport  Port=46  PortDimensions=6
  MC_M2_PZT_M2S7_F(6) [47] : Inport  Port=47  PortDimensions=6
  MC_M2_PZT_M2S1_F(6) [48] : Inport  Port=48  PortDimensions=6
  MC_M2_PZT_M2S2_F(6) [49] : Inport  Port=49  PortDimensions=6
  MC_M2_PZT_M2S3_F(6) [50] : Inport  Port=50  PortDimensions=6
  MC_M2_PZT_M2S4_F(6) [51] : Inport  Port=51  PortDimensions=6
  MC_M2_PZT_M2S5_F(6) [52] : Inport  Port=52  PortDimensions=6
  MC_M2_PZT_M2S6_F(6) [53] : Inport  Port=53  PortDimensions=6
  MC_M2_M2_Hexapod_F(6) [54] : Inport  Port=54  PortDimensions=6
  Build3_SS_PierOSSM1_and_MacrocellM2 : DiscreteStateSpace  A=sysd.sys.A  B=sysd.sys.B  C=sysd.sys.C  D=sysd.sys.D  SampleTime=0.002
  inputs : Mux  Inputs=[3,6,6,6,6,6,6,6,6,6,6,6,6,6,6,6,6,6,6,6,6,6,4,4,4,4,6,6,6,6,3,6,6,6,6,6,6,6,6,6,6,6,6,6,6,6,6,6,6,6,6,6,6,6]
  outputs : Demux  Outputs=[4,4,4,4,6,6,6,6,6,6,6,6,6,6,6,6,6,6,6,6,6,6,42,6,6,6,6,6,6,6,6,6,6,6,6,6,6,4,4,4,4,6,6,6,6,6,6,6,6,6,6,6,42,6,42,42,6,6,6,6,6,6,6,6]
  OSS_AzDrive_top_D(4) [1] : Outport  PortDimensions=4
  OSS_ElDrive_bot_D(4) [2] : Outport  Port=2  PortDimensions=4
  OSS_ElDrive_top_D(4) [3] : Outport  Port=3  PortDimensions=4
  OSS_AzDrive_bot_D(4) [4] : Outport  Port=4  PortDimensions=4
  OSS_TopEnd_6D(6) [5] : Outport  Port=5  PortDimensions=6
  OSS_CRING_6D(6) [6] : Outport  Port=6  PortDimensions=6
  OSS_M2_Hex_D(6) [7] : Outport  Port=7  PortDimensions=6
  OSS_BASE_6D(6) [8] : Outport  Port=8  PortDimensions=6
  OSS_M1S1_HP_cellD(6) [9] : Outport  Port=9  PortDimensions=6
  OSS_M1S2_HP_cellD(6) [10] : Outport  Port=10  PortDimensions=6
  OSS_M1S3_HP_cellD(6) [11] : Outport  Port=11  PortDimensions=6
  OSS_M1S4_HP_cellD(6) [12] : Outport  Port=12  PortDimensions=6
  OSS_M1S5_HP_cellD(6) [13] : Outport  Port=13  PortDimensions=6
  OSS_M1S6_HP_cellD(6) [14] : Outport  Port=14  PortDimensions=6
  OSS_M1S7_HP_cellD(6) [15] : Outport  Port=15  PortDimensions=6
  OSS_M1S1_HP_MirD(6) [16] : Outport  Port=16  PortDimensions=6
  OSS_M1S2_HP_MirD(6) [17] : Outport  Port=17  PortDimensions=6
  OSS_M1S3_HP_MirD(6) [18] : Outport  Port=18  PortDimensions=6
  OSS_M1S4_HP_MirD(6) [19] : Outport  Port=19  PortDimensions=6
  OSS_M1S5_HP_MirD(6) [20] : Outport  Port=20  PortDimensions=6
  OSS_M1S6_HP_MirD(6) [21] : Outport  Port=21  PortDimensions=6
  OSS_M1S7_HP_MirD(6) [22] : Outport  Port=22  PortDimensions=6
  OSS_M1_LOS_6D(42) [23] : Outport  Port=23  PortDimensions=42
  OSS_M1S7_face_6D(6) [24] : Outport  Port=24  PortDimensions=6
  OSS_M1S1_face_6D(6) [25] : Outport  Port=25  PortDimensions=6
  OSS_M1S2_face_6D(6) [26] : Outport  Port=26  PortDimensions=6
  OSS_M1S3_face_6D(6) [27] : Outport  Port=27  PortDimensions=6
  OSS_M1S4_face_6D(6) [28] : Outport  Port=28  PortDimensions=6
  OSS_M1S5_face_6D(6) [29] : Outport  Port=29  PortDimensions=6
  OSS_M1S6_face_6D(6) [30] : Outport  Port=30  PortDimensions=6
  OSS_M1S7_cell_6D(6) [31] : Outport  Port=31  PortDimensions=6
  OSS_M1S1_cell_6D(6) [32] : Outport  Port=32  PortDimensions=6
  OSS_M1S2_cell_6D(6) [33] : Outport  Port=33  PortDimensions=6
  OSS_M1S3_cell_6D(6) [34] : Outport  Port=34  PortDimensions=6
  OSS_M1S4_cell_6D(6) [35] : Outport  Port=35  PortDimensions=6
  OSS_M1S5_cell_6D(6) [36] : Outport  Port=36  PortDimensions=6
  OSS_M1S6_cell_6D(6) [37] : Outport  Port=37  PortDimensions=6
  OSS_AzDrive_top_V(4) [38] : Outport  Port=38  PortDimensions=4
  OSS_ElDrive_bot_V(4) [39] : Outport  Port=39  PortDimensions=4
  OSS_ElDrive_top_V(4) [40] : Outport  Port=40  PortDimensions=4
  OSS_AzDrive_bot_V(4) [41] : Outport  Port=41  PortDimensions=4
  OSS_TopEnd_6V(6) [42] : Outport  Port=42  PortDimensions=6
  OSS_CRING_6V(6) [43] : Outport  Port=43  PortDimensions=6
  OSS_M2_Hex_V(6) [44] : Outport  Port=44  PortDimensions=6
  MC_M2_PZT_M2S7_D(6) [45] : Outport  Port=45  PortDimensions=6
  MC_M2_PZT_M2S1_D(6) [46] : Outport  Port=46  PortDimensions=6
  MC_M2_PZT_M2S2_D(6) [47] : Outport  Port=47  PortDimensions=6
  MC_M2_PZT_M2S3_D(6) [48] : Outport  Port=48  PortDimensions=6
  MC_M2_PZT_M2S4_D(6) [49] : Outport  Port=49  PortDimensions=6
  MC_M2_PZT_M2S5_D(6) [50] : Outport  Port=50  PortDimensions=6
  MC_M2_PZT_M2S6_D(6) [51] : Outport  Port=51  PortDimensions=6
  MC_M2_M2_Hexapod_D(6) [52] : Outport  Port=52  PortDimensions=6
  MC_M2_Cell_6D(42) [53] : Outport  Port=53  PortDimensions=42
  MC_M2_MC_6D(6) [54] : Outport  Port=54  PortDimensions=6
  MC_M2_M2_LOS_6D(42) [55] : Outport  Port=55  PortDimensions=42
  MC_M2_M2_lcl_6D(42) [56] : Outport  Port=56  PortDimensions=42
  MC_M2_PZT_M2S7_V(6) [57] : Outport  Port=57  PortDimensions=6
  MC_M2_PZT_M2S1_V(6) [58] : Outport  Port=58  PortDimensions=6
  MC_M2_PZT_M2S2_V(6) [59] : Outport  Port=59  PortDimensions=6
  MC_M2_PZT_M2S3_V(6) [60] : Outport  Port=60  PortDimensions=6
  MC_M2_PZT_M2S4_V(6) [61] : Outport  Port=61  PortDimensions=6
  MC_M2_PZT_M2S5_V(6) [62] : Outport  Port=62  PortDimensions=6
  MC_M2_PZT_M2S6_V(6) [63] : Outport  Port=63  PortDimensions=6
  MC_M2_M2_Hexapod_V(6) [64] : Outport  Port=64  PortDimensions=6
  wires:
  OSS_Grav_CS0(3) [1]/1 -> inputs/1
  OSS_M1S7_face_6F(6) [2]/1 -> inputs/2
  OSS_M1S1_face_6F(6) [3]/1 -> inputs/3
  OSS_M1S2_face_6F(6) [4]/1 -> inputs/4
  OSS_M1S3_face_6F(6) [5]/1 -> inputs/5
  OSS_M1S4_face_6F(6) [6]/1 -> inputs/6
  OSS_M1S5_face_6F(6) [7]/1 -> inputs/7
  OSS_M1S6_face_6F(6) [8]/1 -> inputs/8
  OSS_M1S7_cell_6F(6) [9]/1 -> inputs/9
  OSS_M1S1_cell_6F(6) [10]/1 -> inputs/10
  OSS_M1S2_cell_6F(6) [11]/1 -> inputs/11
  OSS_M1S3_cell_6F(6) [12]/1 -> inputs/12
  OSS_M1S4_cell_6F(6) [13]/1 -> inputs/13
  OSS_M1S5_cell_6F(6) [14]/1 -> inputs/14
  OSS_M1S6_cell_6F(6) [15]/1 -> inputs/15
  OSS_M1S1_HP_deltaF(6) [16]/1 -> inputs/16
  OSS_M1S2_HP_deltaF(6) [17]/1 -> inputs/17
  OSS_M1S3_HP_deltaF(6) [18]/1 -> inputs/18
  OSS_M1S4_HP_deltaF(6) [19]/1 -> inputs/19
  OSS_M1S5_HP_deltaF(6) [20]/1 -> inputs/20
  OSS_M1S6_HP_deltaF(6) [21]/1 -> inputs/21
  OSS_M1S7_HP_deltaF(6) [22]/1 -> inputs/22
  OSS_AzDrive_top(4) [23]/1 -> inputs/23
  OSS_ElDrive_bot(4) [24]/1 -> inputs/24
  OSS_ElDrive_top(4) [25]/1 -> inputs/25
  OSS_AzDrive_bot(4) [26]/1 -> inputs/26
  OSS_TopEnd_6F(6) [27]/1 -> inputs/27
  OSS_CRING_6F(6) [28]/1 -> inputs/28
  OSS_M2_Hex_F(6) [29]/1 -> inputs/29
  OSS_BASE_6F(6) [30]/1 -> inputs/30
  MC_M2_Grav_CS0(3) [31]/1 -> inputs/31
  MC_M2_Wind6dof_Cell_M2S1(6) [32]/1 -> inputs/32
  MC_M2_Wind6dof_Cell_M2S2(6) [33]/1 -> inputs/33
  MC_M2_Wind6dof_Cell_M2S3(6) [34]/1 -> inputs/34
  MC_M2_Wind6dof_Cell_M2S4(6) [35]/1 -> inputs/35
  MC_M2_Wind6dof_Cell_M2S5(6) [36]/1 -> inputs/36
  MC_M2_Wind6dof_Cell_M2S6(6) [37]/1 -> inputs/37
  MC_M2_Wind6dof_Cell_M2S7(6) [38]/1 -> inputs/38
  MC_M2_Wind6dof_MacroCell(6) [39]/1 -> inputs/39
  MC_M2_Wind6dof_Mir_M2S7(6) [40]/1 -> inputs/40
  MC_M2_Wind6dof_Mir_M2S1(6) [41]/1 -> inputs/41
  MC_M2_Wind6dof_Mir_M2S2(6) [42]/1 -> inputs/42
  MC_M2_Wind6dof_Mir_M2S3(6) [43]/1 -> inputs/43
  MC_M2_Wind6dof_Mir_M2S4(6) [44]/1 -> inputs/44
  MC_M2_Wind6dof_Mir_M2S5(6) [45]/1 -> inputs/45
  MC_M2_Wind6dof_Mir_M2S6(6) [46]/1 -> inputs/46
  MC_M2_PZT_M2S7_F(6) [47]/1 -> inputs/47
  MC_M2_PZT_M2S1_F(6) [48]/1 -> inputs/48
  MC_M2_PZT_M2S2_F(6) [49]/1 -> inputs/49
  MC_M2_PZT_M2S3_F(6) [50]/1 -> inputs/50
  MC_M2_PZT_M2S4_F(6) [51]/1 -> inputs/51
  MC_M2_PZT_M2S5_F(6) [52]/1 -> inputs/52
  MC_M2_PZT_M2S6_F(6) [53]/1 -> inputs/53
  MC_M2_M2_Hexapod_F(6) [54]/1 -> inputs/54
  inputs/1 -> Build3_SS_PierOSSM1_and_MacrocellM2/1
  Build3_SS_PierOSSM1_and_MacrocellM2/1 -> outputs/1
  outputs/1 -> OSS_AzDrive_top_D(4) [1]/1
  outputs/2 -> OSS_ElDrive_bot_D(4) [2]/1
  outputs/3 -> OSS_ElDrive_top_D(4) [3]/1
  outputs/4 -> OSS_AzDrive_bot_D(4) [4]/1
  outputs/5 -> OSS_TopEnd_6D(6) [5]/1
  outputs/6 -> OSS_CRING_6D(6) [6]/1
  outputs/7 -> OSS_M2_Hex_D(6) [7]/1
  outputs/8 -> OSS_BASE_6D(6) [8]/1
  outputs/9 -> OSS_M1S1_HP_cellD(6) [9]/1
  outputs/10 -> OSS_M1S2_HP_cellD(6) [10]/1
  outputs/11 -> OSS_M1S3_HP_cellD(6) [11]/1
  outputs/12 -> OSS_M1S4_HP_cellD(6) [12]/1
  outputs/13 -> OSS_M1S5_HP_cellD(6) [13]/1
  outputs/14 -> OSS_M1S6_HP_cellD(6) [14]/1
  outputs/15 -> OSS_M1S7_HP_cellD(6) [15]/1
  outputs/16 -> OSS_M1S1_HP_MirD(6) [16]/1
  outputs/17 -> OSS_M1S2_HP_MirD(6) [17]/1
  outputs/18 -> OSS_M1S3_HP_MirD(6) [18]/1
  outputs/19 -> OSS_M1S4_HP_MirD(6) [19]/1
  outputs/20 -> OSS_M1S5_HP_MirD(6) [20]/1
  outputs/21 -> OSS_M1S6_HP_MirD(6) [21]/1
  outputs/22 -> OSS_M1S7_HP_MirD(6) [22]/1
  outputs/23 -> OSS_M1_LOS_6D(42) [23]/1
  outputs/24 -> OSS_M1S7_face_6D(6) [24]/1
  outputs/25 -> OSS_M1S1_face_6D(6) [25]/1
  outputs/26 -> OSS_M1S2_face_6D(6) [26]/1
  outputs/27 -> OSS_M1S3_face_6D(6) [27]/1
  outputs/28 -> OSS_M1S4_face_6D(6) [28]/1
  outputs/29 -> OSS_M1S5_face_6D(6) [29]/1
  outputs/30 -> OSS_M1S6_face_6D(6) [30]/1
  outputs/31 -> OSS_M1S7_cell_6D(6) [31]/1
  outputs/32 -> OSS_M1S1_cell_6D(6) [32]/1
  outputs/33 -> OSS_M1S2_cell_6D(6) [33]/1
  outputs/34 -> OSS_M1S3_cell_6D(6) [34]/1
  outputs/35 -> OSS_M1S4_cell_6D(6) [35]/1
  outputs/36 -> OSS_M1S5_cell_6D(6) [36]/1
  outputs/37 -> OSS_M1S6_cell_6D(6) [37]/1
  outputs/38 -> OSS_AzDrive_top_V(4) [38]/1
  outputs/39 -> OSS_ElDrive_bot_V(4) [39]/1
  outputs/40 -> OSS_ElDrive_top_V(4) [40]/1
  outputs/41 -> OSS_AzDrive_bot_V(4) [41]/1
  outputs/42 -> OSS_TopEnd_6V(6) [42]/1
  outputs/43 -> OSS_CRING_6V(6) [43]/1
  outputs/44 -> OSS_M2_Hex_V(6) [44]/1
  outputs/45 -> MC_M2_PZT_M2S7_D(6) [45]/1
  outputs/46 -> MC_M2_PZT_M2S1_D(6) [46]/1
  outputs/47 -> MC_M2_PZT_M2S2_D(6) [47]/1
  outputs/48 -> MC_M2_PZT_M2S3_D(6) [48]/1
  outputs/49 -> MC_M2_PZT_M2S4_D(6) [49]/1
  outputs/50 -> MC_M2_PZT_M2S5_D(6) [50]/1
  outputs/51 -> MC_M2_PZT_M2S6_D(6) [51]/1
  outputs/52 -> MC_M2_M2_Hexapod_D(6) [52]/1
  outputs/53 -> MC_M2_Cell_6D(42) [53]/1
  outputs/54 -> MC_M2_MC_6D(6) [54]/1
  outputs/55 -> MC_M2_M2_LOS_6D(42) [55]/1
  outputs/56 -> MC_M2_M2_lcl_6D(42) [56]/1
  outputs/57 -> MC_M2_PZT_M2S7_V(6) [57]/1
  outputs/58 -> MC_M2_PZT_M2S1_V(6) [58]/1
  outputs/59 -> MC_M2_PZT_M2S2_V(6) [59]/1
  outputs/60 -> MC_M2_PZT_M2S3_V(6) [60]/1
  outputs/61 -> MC_M2_PZT_M2S4_V(6) [61]/1
  outputs/62 -> MC_M2_PZT_M2S5_V(6) [62]/1
  outputs/63 -> MC_M2_PZT_M2S6_V(6) [63]/1
  outputs/64 -> MC_M2_M2_Hexapod_V(6) [64]/1

== system AcO_Ctrl_Geometric_headless_R2016a/Structural Dynamics V3.3/Structural Dynamics V3.5.2/Structural Dynamics Plus CL Az El M1 force/Az Control ==
  AverageAzDisp : Inport
  Azimuth Controller : DiscreteFilter  Numerator=Az_C.num{1}  Denominator=Az_C.den{1}  SampleTime=1/500
  DistributeForce : Gain  Gain=[-ones(4,1);ones(4,1)]  Multiplication=Matrix(K*u)
  AzForces : Outport
  wires:
  AverageAzDisp/1 -> Azimuth Controller/1
  DistributeForce/1 -> AzForces/1
  Azimuth Controller/1 -> DistributeForce/1

== system AcO_Ctrl_Geometric_headless_R2016a/Structural Dynamics V3.3/Structural Dynamics V3.5.2/Structural Dynamics Plus CL Az El M1 force/Az El Sensing ==
  note: Note: units are m, not radians for these loops!
      | These loops delta the top and bottom displacements in tangential direction, and average the results.
  Az_disp(8) : Inport
  El_disp(8) : Inport  Port=2
  GIR_disp(4) : Inport  Port=3
  Az : Scope
  Demux : Demux  Outputs=[4,4]
  Demux1 : Demux  Outputs=[4,4]
  Demux2 : Demux  Outputs=[2,2]
  El : Scope
  GIR : Scope
  Sum1 : Sum  Inputs=-+|
  Sum2 : Sum  Inputs=-+|
  Sum3 : Sum  Inputs=-+|
  average : Gain  Gain=ones(1,4)/4  Multiplication=Matrix(K*u)
  average1 : Gain  Gain=ones(1,4)/4  Multiplication=Matrix(K*u)
  average2 : Gain  Gain=ones(1,2)/2  Multiplication=Matrix(K*u)
  El_average(1) : Outport
  Az_average(1) : Outport  Port=2
  GIR_average(1) : Outport  Port=3
  wires:
  average/1 -> El/1, El_average(1)/1
  average1/1 -> Az_average(1)/1, Az/1
  Sum3/1 -> average1/1
  Sum2/1 -> average/1
  Az_disp(8)/1 -> Demux/1
  Demux/2 -> Sum3/2
  Demux/1 -> Sum3/1
  El_disp(8)/1 -> Demux1/1
  Demux1/1 -> Sum2/1
  Demux1/2 -> Sum2/2
  average2/1 -> GIR_average(1)/1, GIR/1
  Sum1/1 -> average2/1
  GIR_disp(4)/1 -> Demux2/1
  Demux2/1 -> Sum1/1
  Demux2/2 -> Sum1/2

== system AcO_Ctrl_Geometric_headless_R2016a/Structural Dynamics V3.3/Structural Dynamics V3.5.2/Structural Dynamics Plus CL Az El M1 force/El Control ==
  AverageElDisp : Inport
  DistributeForces : Gain  Gain=[-ones(4,1);ones(4,1)]  Multiplication=Matrix(K*u)
  Elevation Controller : DiscreteFilter  Numerator=El_C.num{1}  Denominator=El_C.den{1}  SampleTime=1/500
  ElForces : Outport
  wires:
  Elevation Controller/1 -> DistributeForces/1
  DistributeForces/1 -> ElForces/1
  AverageElDisp/1 -> Elevation Controller/1
